simulink model "sl_drivepoint"  (Simulink 7.6)
settings: Solver=ode45  StartTime=0.0  StopTime=15.0  RelTol=1e-3
undefined symbols (not defined in the file or in its folder): xg
libraries: roblocks x2, simulink x1
settings Model: Creator=pic  LastModifiedBy=n6334687
settings DataIOCC: LimitDataPoints=off  ReturnWorkspaceOutputs=on
settings DebuggingCC: StrictBusMsg=Warning

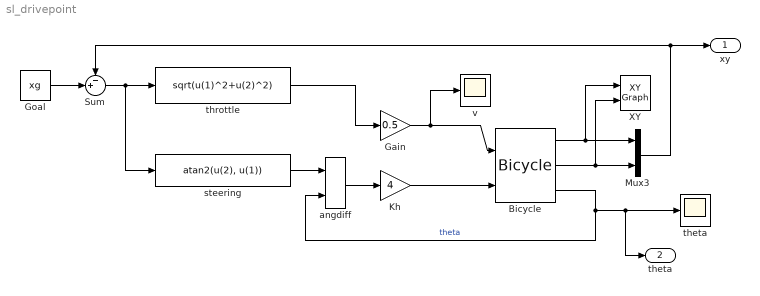
== system sl_drivepoint ==
  Bicycle : roblocks/Dynamics/Bicycle  SystemSampleTime=-1  accel=1  vlim=1  alim=2  x0=x0  handbrake=0
  Gain : Gain  Gain=0.5
  Goal : Constant  Value=xg
  Kh : Gain  Gain=4
  Mux3 : Mux  Inputs=2
  Sum : Sum  Inputs=-+|
  XY : simulink/Sinks/XY Graph  SystemSampleTime=-1  xmin=0  xmax=10  ymin=0  ymax=10  st=-1
  angdiff : roblocks/angdiff  SystemSampleTime=-1
  steering : Fcn  Expr=atan2(u(2), u(1))
  theta : Scope
  throttle : Fcn  Expr=sqrt(u(1)^2+u(2)^2)
  v : Scope
  xy : Outport
  "theta " : Outport  Port=2
  wires:
  Bicycle/1 -> Mux3/1, XY/1
  Bicycle/2 -> Mux3/2, XY/2
  Mux3/1 -> xy/1, Sum/1
  Sum/1 -> throttle/1, steering/1
  throttle/1 -> Gain/1
  steering/1 -> angdiff/1
  Bicycle/3 -> theta/1, "theta "/1, angdiff/2  "theta"
  angdiff/1 -> Kh/1
  Gain/1 -> v/1, Bicycle/1
  Goal/1 -> Sum/2
  Kh/1 -> Bicycle/2
